simulink model "Partage_Simulink_2013"  (Simulink 8.2)
settings: Solver=ode5  SolverMode=SingleTasking  StartTime=0.0  StopTime=Smax/v-1  FixedStep=0.02  RelTol=1e-3
values from neighbouring files (symbols this model uses):
  A = eye(3) + A*Ts    [funcDriverModelAblamvi.m]    (also in funcDriverModelLoauy.m; funcNeuromuscularModel.m; funcTwoPointsVisualModel.m)
  alpha = 0.6    [Tref_combined.m]
  Aw = [-1/tau   1/tau ... (first row only)    [Tref_combined.m]
  Bs = 5.7    [Tref_combined.m]
  C = [       0       0       1       ]    [funcDriverModelAblamvi.m]    (also in funcDriverModelLoauy.m = zeros(2,3); funcNeuromuscularModel.m = zeros(1,1); funcTwoPointsVisualModel.m = zeros(1,2))
  Cw = [1  0]    [Tref_combined.m]
  EX0 = route.EX0    [Tref_combined.m]
  EY0 = route.EY0    [Tref_combined.m]
  F = A11d-L1*A21d    [Tref_combined.m]
  G = F*L1+A12d-L1*A22d    [Tref_combined.m]
  H = B1d-L1*B2d    [Tref_combined.m]
  Is = 0.05    [Tref_combined.m]
  Kplus_deltad = polyfit(alpha_vec,Kplus_vec(4,:),6)    [Tref_combined.m]
  Kplus_psiL = polyfit(alpha_vec,Kplus_vec(2,:),6)    [Tref_combined.m]
  Kplus_r = polyfit(alpha_vec,Kplus_vec(1,:),6)    [Tref_combined.m]
  Kplus_yL = polyfit(alpha_vec,Kplus_vec(3,:),7)    [Tref_combined.m]
  L1 = place(A11d',A21d',3*P0)'    [Tref_combined.m]
  Lo = acker(Aw',Cw',3*E)'    [Tref_combined.m]
  sw_DR = 1    [Tref_combined.m]
  sw_LQ = 0    [Tref_combined.m]
  T_horizon = 2    [Tref_combined.m]
  v = 18    [DriverModelLouayEstimationByPEM.m]    (also in NeuromuscularModelEstimationByPEM.m = 17; ParameterEstimationByPEM.m; Tref_combined.m; TwoPointsVisualModelEstimationByPEM.m = 17)
undefined symbols (not defined in the file or in its folder): Abic, Ad, At, Avr, B1, B1t, B2, B2t, Bbic, Bd, Bvr, Cbic, Cvr, D2, Dbic, Dvr, EPHI0, F2_a, fai_0_a, fai_2T8_a, fai_3T8_a, fai_4T8_a, fai_5T8_a, fai_6T8_a, fai_7T8_a, fai_T8_a, fai_T_a, Kplus_a, Measure, Measure_combined
libraries: simulink x2
settings Model: Creator=user  LastModifiedBy=Yishen Zhao
settings OptimizationCC: InitFltsAndDblsToZero=on
settings DebuggingCC: SaveWithParameterizedLinksMsg=none  SignalResolutionControl=TryResolveAllWithWarning  SolverPrmCheckMsg=none  MultiTaskDSMMsg=warning  MultiTaskCondExecSysMsg=none  FcnCallInpInsideContextMsg=EnableAllAsWarning  FrameProcessingCompatibilityMsg=error
settings GRTTargetCC: TargetFcnLib=ansi_tfl_tmw.mat  CodeReplacementLibrary=C89/C90 (ANSI)

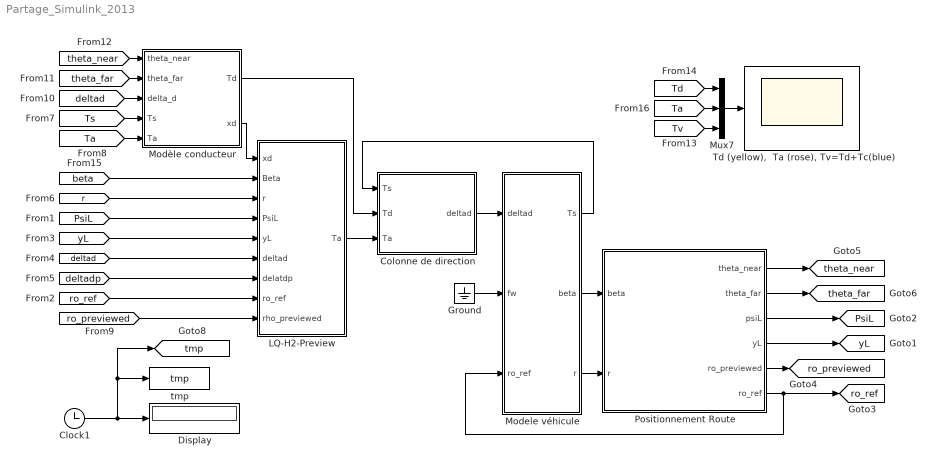
== system Partage_Simulink_2013 ==
  Clock1 : Clock
      settings: Decimation=60
  Colonne de direction : Subsystem
  Display : Display
  Ground : Ground
  LQ-H2-Preview : Subsystem
  Modele véhicule : Subsystem
  Modèle conducteur : Subsystem
  Mux7 : Mux  Inputs=3
  Positionnement Route : Subsystem  mask(Calcul des coordonnées x et y){}
      mask Display: disp('Calcul des coordonnées')
  "Td (yellow),  Ta (rose), Tv=Td+Tc(blue)" : Scope
      settings: TimeRange=auto  MaxDataPoints=5000  SaveName=TdTcTv  YMin=-20  YMax=15  SampleTime=-1
  tmp : ToWorkspace  VariableName=tmp  SampleTime=-1
  tag scope: PsiL=global, ro_previewed=global, ro_ref=global, theta_far=global, theta_near=global, tmp=global, yL=global
  wires:
  Clock1/1 -> Display/1, tmp/1, [tmp]
  Modele véhicule/3(r) -> Positionnement Route/2(r)
  Colonne de direction/1(deltad) -> Modele véhicule/1(deltad)
  Positionnement Route/6(ro_ref) -> [ro_ref], Modele véhicule/3(ro_ref)
  [r] -> LQ-H2-Preview/3(r)
  [PsiL] -> LQ-H2-Preview/4(PsiL)
  [yL] -> LQ-H2-Preview/5(yL)
  [deltad] -> LQ-H2-Preview/6(deltad)
  [deltadp] -> LQ-H2-Preview/7(delatdp)
  [ro_ref] -> LQ-H2-Preview/8(ro_ref)
  Positionnement Route/5(ro_previewed) -> [ro_previewed]
  Positionnement Route/1(theta_near) -> [theta_near]
  Positionnement Route/2(theta_far) -> [theta_far]
  [deltad] -> Modèle conducteur/3(delta_d)
  Positionnement Route/4(yL) -> [yL]
  Positionnement Route/3(psiL) -> [PsiL]
  Modele véhicule/2(beta) -> Positionnement Route/1(beta)
  Modele véhicule/1(Ts) -> Colonne de direction/1(Ts)
  [beta] -> LQ-H2-Preview/2(Beta)
  Modèle conducteur/2(xd) -> LQ-H2-Preview/1(xd)
  Mux7/1 -> "Td (yellow),  Ta (rose), Tv=Td+Tc(blue)"/1
  [theta_near] -> Modèle conducteur/1(theta_near)
  [Ts] -> Modèle conducteur/4(Ts)
  [Ta] -> Modèle conducteur/5(Ta)
  [theta_far] -> Modèle conducteur/2(theta_far)
  Ground/1 -> Modele véhicule/2(fw)
  [Td] -> Mux7/1
  [Ta] -> Mux7/2
  [Tv] -> Mux7/3
  Modèle conducteur/1(Td) -> Colonne de direction/2(Td)
  LQ-H2-Preview/1(Ta) -> Colonne de direction/3(Ta)
  [ro_previewed] -> LQ-H2-Preview/9(rho_previewed)

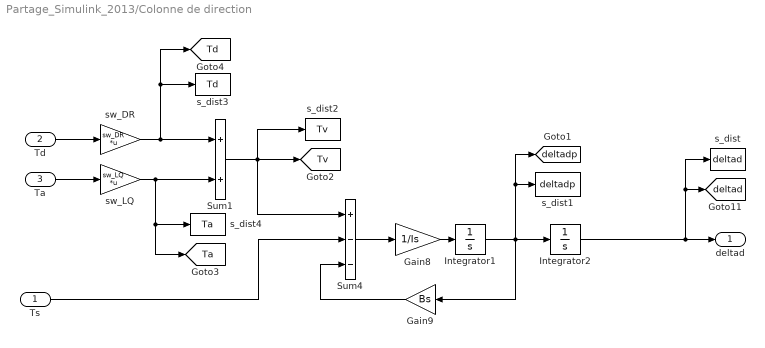
== system Partage_Simulink_2013/Colonne de direction ==
  Ts : Inport
  Td : Inport  Port=2
  Ta : Inport  Port=3
  Gain8 : Gain  Gain=1/Is  SaturateOnIntegerOverflow=on  OutDataTypeStr=Inherit: Same as input  ParamDataTypeStr=Inherit: Same as input
  Gain9 : Gain  Gain=Bs  SaturateOnIntegerOverflow=on  OutDataTypeStr=Inherit: Same as input  ParamDataTypeStr=Inherit: Same as input
  Integrator1 : Integrator
  Integrator2 : Integrator
  Sum1 : Sum  SaturateOnIntegerOverflow=on  InputSameDT=on  OutDataTypeStr=Inherit: Same as first input
  Sum4 : Sum  Inputs=+--  SaturateOnIntegerOverflow=on  InputSameDT=on  OutDataTypeStr=Inherit: Same as first input
  s_dist : ToWorkspace  VariableName=deltad  SampleTime=-1
  s_dist1 : ToWorkspace  VariableName=deltadp  SampleTime=-1
  s_dist2 : ToWorkspace  VariableName=Tv  SampleTime=-1
  s_dist3 : ToWorkspace  VariableName=Td  SampleTime=-1
  s_dist4 : ToWorkspace  VariableName=Ta  SampleTime=-1
  sw_DR : Gain  Gain=sw_DR  Multiplication=Matrix(K*u)  SaturateOnIntegerOverflow=on  OutDataTypeStr=Inherit: Same as input  ParamDataTypeStr=Inherit: Same as input
  sw_LQ : Gain  Gain=sw_LQ  Multiplication=Matrix(K*u)  SaturateOnIntegerOverflow=on  OutDataTypeStr=Inherit: Same as input  ParamDataTypeStr=Inherit: Same as input
  deltad : Outport
  tag scope: Ta=global, Td=global, Tv=global, deltad=global, deltadp=global
  wires:
  Gain8/1 -> Integrator1/1
  Sum4/1 -> Gain8/1
  Integrator1/1 -> Integrator2/1, s_dist1/1, [deltadp], Gain9/1
  Integrator2/1 -> deltad/1, [deltad], s_dist/1
  Ta/1 -> sw_LQ/1
  Gain9/1 -> Sum4/3
  Td/1 -> sw_DR/1
  sw_DR/1 -> Sum1/1, s_dist3/1, [Td]
  Ts/1 -> Sum4/2
  Sum1/1 -> Sum4/1, [Tv], s_dist2/1
  sw_LQ/1 -> s_dist4/1, [Ta], Sum1/2

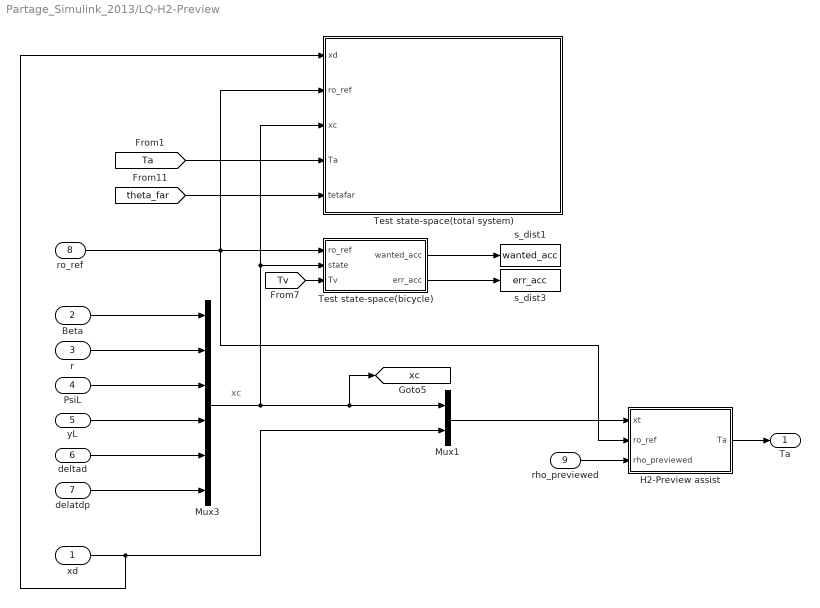
== system Partage_Simulink_2013/LQ-H2-Preview ==
  note: xc
  xd : Inport
  Beta : Inport  Port=2
  r : Inport  Port=3
  PsiL : Inport  Port=4
  yL : Inport  Port=5
  deltad : Inport  Port=6
  delatdp : Inport  Port=7
  ro_ref : Inport  Port=8
  rho_previewed : Inport  Port=9
  H2-Preview assist : Subsystem
  Mux1 : Mux  Inputs=2
  Mux3 : Mux  Inputs=6
  "Test state-space(bicycle) " : Subsystem
  Test state-space(total system) : Subsystem
  s_dist1 : ToWorkspace  VariableName=wanted_acc  SampleTime=-1
  s_dist3 : ToWorkspace  VariableName=err_acc  SampleTime=-1
  Ta : Outport
  tag scope: xc=global
  wires:
  Mux3/1 -> Test state-space(total system)/3(xc), "Test state-space(bicycle) "/2(state), [xc], Mux1/1
  Beta/1 -> Mux3/1
  r/1 -> Mux3/2
  PsiL/1 -> Mux3/3
  yL/1 -> Mux3/4
  deltad/1 -> Mux3/5
  delatdp/1 -> Mux3/6
  "Test state-space(bicycle) "/1(wanted_acc) -> s_dist1/1
  "Test state-space(bicycle) "/2(err_acc) -> s_dist3/1
  [Tv] -> "Test state-space(bicycle) "/3(Tv)
  [theta_far] -> Test state-space(total system)/5(tetafar)
  xd/1 -> Test state-space(total system)/1(xd), Mux1/2
  ro_ref/1 -> H2-Preview assist/2("ro_ref "), "Test state-space(bicycle) "/1(ro_ref), Test state-space(total system)/2(ro_ref)
  Mux1/1 -> H2-Preview assist/1(xt)
  [Ta] -> Test state-space(total system)/4(Ta)
  H2-Preview assist/1(Ta) -> Ta/1
  rho_previewed/1 -> H2-Preview assist/3(rho_previewed)

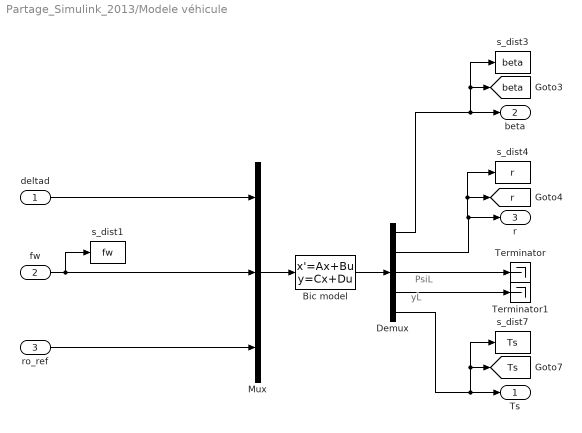
== system Partage_Simulink_2013/Modele véhicule ==
  note: PsiL
  note: yL
  deltad : Inport
  fw : Inport  Port=2
  ro_ref : Inport  Port=3
  Bic model : StateSpace  A=Abic  B=Bbic  C=Cbic  D=Dbic  X0=[0;0;0;0]
  Demux : Demux  Outputs=5
  Mux : Mux  Inputs=3
  Terminator : Terminator
  Terminator1 : Terminator
  s_dist1 : ToWorkspace  VariableName=fw  SampleTime=-1
  s_dist3 : ToWorkspace  VariableName=beta  SampleTime=-1
  s_dist4 : ToWorkspace  VariableName=r  SampleTime=-1
  s_dist7 : ToWorkspace  VariableName=Ts  SampleTime=-1
  Ts : Outport
  beta : Outport  Port=2
  r : Outport  Port=3
  tag scope: Ts=global, beta=global, r=global
  wires:
  fw/1 -> Mux/2, s_dist1/1
  ro_ref/1 -> Mux/3
  Mux/1 -> Bic model/1
  Bic model/1 -> Demux/1
  deltad/1 -> Mux/1
  Demux/1 -> beta/1, [beta], s_dist3/1
  Demux/2 -> s_dist4/1, [r], r/1
  Demux/5 -> Ts/1, [Ts], s_dist7/1
  Demux/3 -> Terminator/1
  Demux/4 -> Terminator1/1

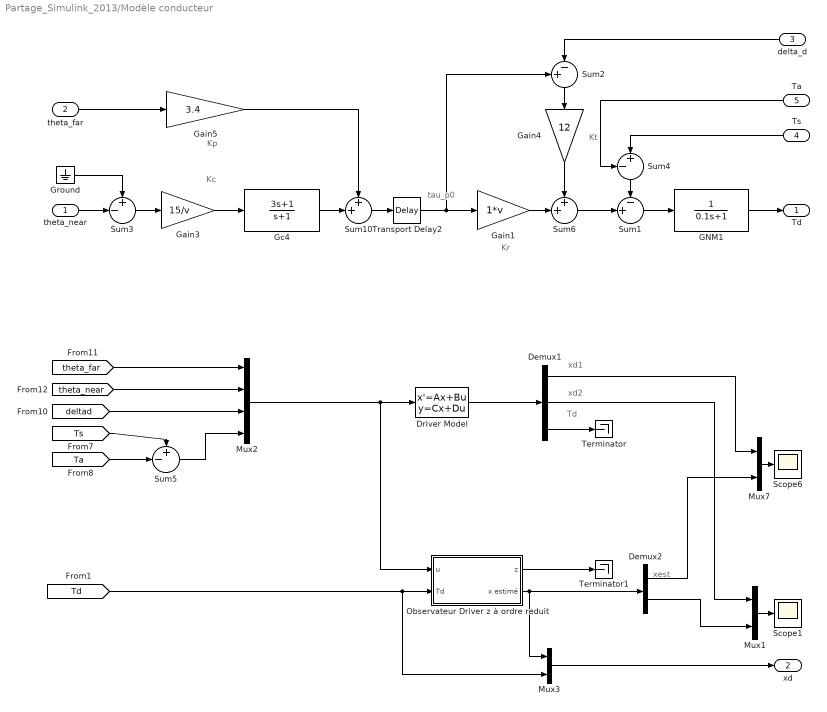
== system Partage_Simulink_2013/Modèle conducteur ==
  note: Kc
  note: tau_p0
  note: Kr
  note: Kp
  note: Kt
  note: xd1
  note: xd2
  note: Td
  note: xest
  theta_near : Inport
  theta_far : Inport  Port=2
  delta_d : Inport  Port=3
  Ts : Inport  Port=4
  Ta : Inport  Port=5
  Demux1 : Demux  Outputs=3
  Demux2 : Demux  Outputs=2
  Driver Model : StateSpace  A=Ad  B=Bd  C=[1 0 0;0 1 0;0 0 1]  D=[0 0 0 0;0 0 0 0;0 0 0 0]  X0=[0;0;0]
  GNM1 : TransferFcn  Numerator=1  Denominator=[0.1 1]
  Gain1 : Gain  Gain=1*v  SaturateOnIntegerOverflow=on  OutDataTypeStr=Inherit: Same as input  ParamDataTypeStr=Inherit: Same as input
  Gain3 : Gain  Gain=15/v  SaturateOnIntegerOverflow=on  OutDataTypeStr=Inherit: Same as input  ParamDataTypeStr=Inherit: Same as input
  Gain4 : Gain  Gain=12  SaturateOnIntegerOverflow=on  OutDataTypeStr=Inherit: Same as input  ParamDataTypeStr=Inherit: Same as input
  Gain5 : Gain  Gain=3.4  SaturateOnIntegerOverflow=on  OutDataTypeStr=Inherit: Same as input  ParamDataTypeStr=Inherit: Same as input
  Gc4 : TransferFcn  Numerator=[3 1]  Denominator=[1 1]
  Ground : Ground
  Mux1 : Mux  Inputs=2
  Mux2 : Mux
  Mux3 : Mux  Inputs=2
  Mux7 : Mux  Inputs=2
  Observateur Driver z à ordre reduit : Subsystem
  Scope1 : Scope
      settings: TimeRange=auto  LimitDataPoints=on  MaxDataPoints=5000  SaveToWorkspace=off  SaveName=ScopeData9  YMin=-8  YMax=7  SampleTime=-1
  Scope6 : Scope
      settings: TimeRange=auto  LimitDataPoints=on  MaxDataPoints=5000  SaveToWorkspace=off  SaveName=ScopeData8  YMin=-0.15  YMax=0.2  SampleTime=-1
  Sum1 : Sum  Inputs=-+|  SaturateOnIntegerOverflow=on  InputSameDT=on  OutDataTypeStr=Inherit: Same as first input
  Sum10 : Sum  Inputs=++|  SaturateOnIntegerOverflow=on  InputSameDT=on  OutDataTypeStr=Inherit: Same as first input
  Sum2 : Sum  Inputs=+-|  SaturateOnIntegerOverflow=on  InputSameDT=on  OutDataTypeStr=Inherit: Same as first input
  Sum3 : Sum  Inputs=+-|  SaturateOnIntegerOverflow=on  InputSameDT=on  OutDataTypeStr=Inherit: Same as first input
  Sum4 : Sum  Inputs=-+|  SaturateOnIntegerOverflow=on  InputSameDT=on  OutDataTypeStr=Inherit: Same as first input
  Sum5 : Sum  Inputs=+-|  SaturateOnIntegerOverflow=on  InputSameDT=on  OutDataTypeStr=Inherit: Same as first input
  Sum6 : Sum  Inputs=++|  SaturateOnIntegerOverflow=on  InputSameDT=on  OutDataTypeStr=Inherit: Same as first input
  Terminator : Terminator
  Terminator1 : Terminator
  Transport Delay2 : TransportDelay  DelayTime=0.04
  Td : Outport
  xd : Outport  Port=2
  wires:
  theta_far/1 -> Gain5/1
  theta_near/1 -> Sum3/2
  Ground/1 -> Sum3/1
  Gain5/1 -> Sum10/1
  Sum3/1 -> Gain3/1
  Sum1/1 -> GNM1/1
  Gain3/1 -> Gc4/1
  Gc4/1 -> Sum10/2
  Sum10/1 -> Transport Delay2/1
  Transport Delay2/1 -> Sum2/1, Gain1/1
  Gain1/1 -> Sum6/2
  delta_d/1 -> Sum2/2
  Sum2/1 -> Gain4/1
  Gain4/1 -> Sum6/1
  Driver Model/1 -> Demux1/1
  [theta_near] -> Mux2/2
  [deltad] -> Mux2/3
  GNM1/1 -> Td/1
  Sum6/1 -> Sum1/2
  Sum5/1 -> Mux2/4
  [Ta] -> Sum5/2
  [Ts] -> Sum5/1
  Sum4/1 -> Sum1/1
  Ts/1 -> Sum4/2
  Ta/1 -> Sum4/1
  [theta_far] -> Mux2/1
  Observateur Driver z à ordre reduit/2(x estimé) -> Demux2/1, Mux3/1
  Mux7/1 -> Scope6/1
  Demux1/1 -> Mux7/1
  Demux2/1 -> Mux7/2
  Mux1/1 -> Scope1/1
  Demux1/2 -> Mux1/1
  Demux2/2 -> Mux1/2
  [Td] -> Observateur Driver z à ordre reduit/2(Td), Mux3/2
  Mux2/1 -> Driver Model/1, Observateur Driver z à ordre reduit/1(u)
  Mux3/1 -> xd/1
  Demux1/3 -> Terminator/1
  Observateur Driver z à ordre reduit/1(z) -> Terminator1/1

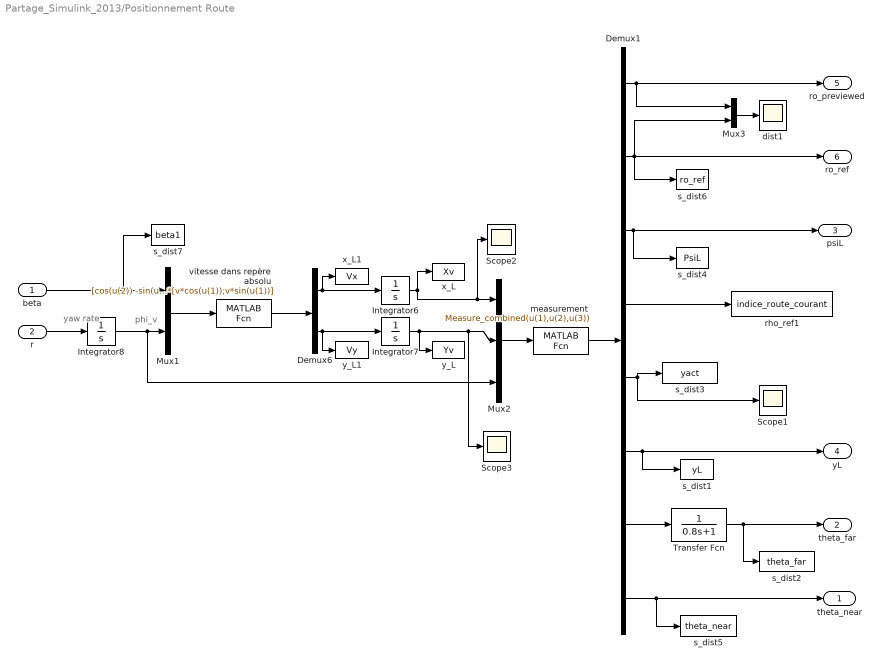
== system Partage_Simulink_2013/Positionnement Route ==
  note: phi_v
  note: yaw rate
  beta : Inport
  r : Inport  Port=2
  Demux1 : Demux  Outputs=8
  Demux6 : Demux  Outputs=2
  Integrator6 : Integrator  InitialCondition=EX0
  Integrator7 : Integrator  InitialCondition=EY0
  Integrator8 : Integrator  InitialCondition=EPHI0
  Mux1 : Mux  Inputs=2
  Mux2 : Mux  Inputs=3
  Mux3 : Mux  Inputs=2
  Scope1 : Scope
      settings: TimeRange=auto  LimitDataPoints=on  MaxDataPoints=5000  SaveToWorkspace=off  SaveName=ScopeData7  YMin=-4.92978  YMax=4.87495  SampleTime=-1
  Scope2 : Scope
      settings: TimeRange=auto  LimitDataPoints=on  MaxDataPoints=5000  SaveToWorkspace=off  SaveName=ScopeData18  YMin=-967.24148  YMax=375.02741  SampleTime=-1
  Scope3 : Scope
      settings: TimeRange=auto  LimitDataPoints=on  MaxDataPoints=5000  SaveToWorkspace=off  SaveName=ScopeData19  YMin=-10  YMax=10  SampleTime=-1
  Transfer Fcn : TransferFcn  Denominator=[0.8 1]
  dist1 : Scope
      settings: TimeRange=auto  MaxDataPoints=5000  SaveToWorkspace=off  SaveName=ScopeData10  YMin=-0.03  YMax=0.04  SampleTime=-1
  measurement : MATLABFcn  MATLABFcn=Measure_combined(u(1),u(2),u(3))  OutputDimensions=8
  rho_ref1 : ToWorkspace  VariableName=indice_route_courant  SampleTime=-1
  s_dist1 : ToWorkspace  VariableName=yL  SampleTime=-1
  s_dist2 : ToWorkspace  VariableName=theta_far  SampleTime=-1
  s_dist3 : ToWorkspace  VariableName=yact  SampleTime=-1
  s_dist4 : ToWorkspace  VariableName=PsiL  SampleTime=-1
  s_dist5 : ToWorkspace  VariableName=theta_near  SampleTime=-1
  s_dist6 : ToWorkspace  VariableName=ro_ref  SampleTime=-1
  s_dist7 : ToWorkspace  VariableName=beta1  SampleTime=-1
  vitesse dans repère absolu : MATLABFcn  MATLABFcn=[cos(u(2)) -sin(u(2));sin(u(2)) cos(u(2)) ]*[v*cos(u(1));v*sin(u(1))]  OutputDimensions=2
  x_L : ToWorkspace  VariableName=Xv  SampleTime=-1
  x_L1 : ToWorkspace  VariableName=Vx  SampleTime=-1
  y_L : ToWorkspace  VariableName=Yv  SampleTime=-1
  y_L1 : ToWorkspace  VariableName=Vy  SampleTime=-1
  theta_near : Outport
  theta_far : Outport  Port=2
  psiL : Outport  Port=3
  yL : Outport  Port=4
  ro_previewed : Outport  Port=5
  ro_ref : Outport  Port=6
  wires:
  vitesse dans repère absolu/1 -> Demux6/1
  Integrator8/1 -> Mux1/2, Mux2/3
  Mux1/1 -> vitesse dans repère absolu/1
  Demux6/1 -> Integrator6/1, x_L1/1
  Demux6/2 -> y_L1/1, Integrator7/1
  Integrator6/1 -> Scope2/1, Mux2/1, x_L/1
  Integrator7/1 -> Scope3/1, Mux2/2, y_L/1
  Mux2/1 -> measurement/1
  r/1 -> Integrator8/1
  Demux1/1 -> ro_previewed/1, Mux3/1
  Demux1/2 -> ro_ref/1, s_dist6/1, Mux3/2
  measurement/1 -> Demux1/1
  Demux1/4 -> rho_ref1/1
  Demux1/5 -> s_dist3/1, Scope1/1
  Demux1/8 -> s_dist5/1, theta_near/1
  Demux1/7 -> Transfer Fcn/1
  Demux1/3 -> s_dist4/1, psiL/1
  Demux1/6 -> s_dist1/1, yL/1
  Transfer Fcn/1 -> s_dist2/1, theta_far/1
  Mux3/1 -> dist1/1
  beta/1 -> s_dist7/1, Mux1/1

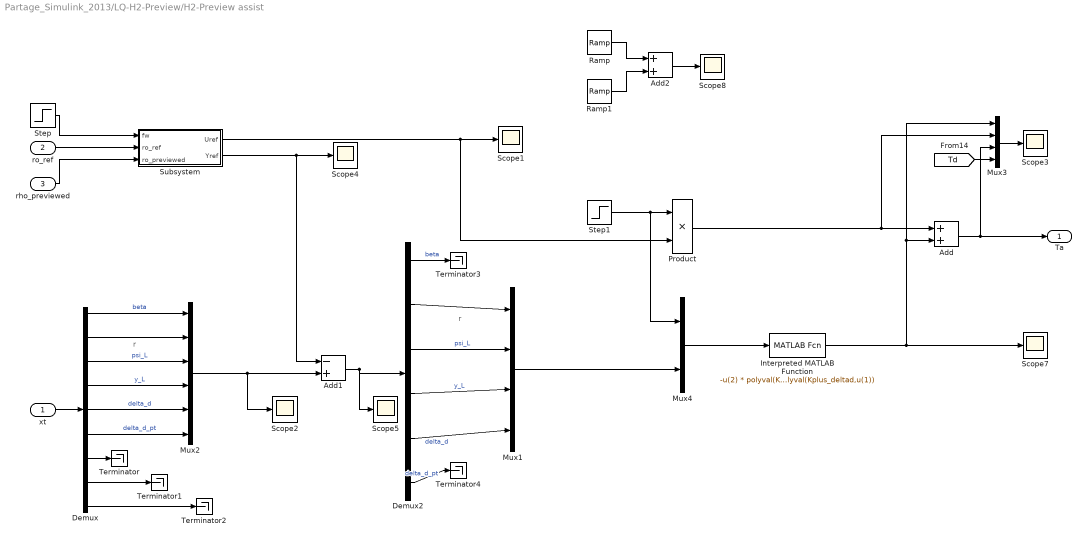
== system Partage_Simulink_2013/LQ-H2-Preview/H2-Preview assist ==
  note: r
  note: r
  xt : Inport
  "ro_ref " : Inport  Port=2
  rho_previewed : Inport  Port=3
  Add : Sum
  Add1 : Sum  Inputs=-+
  Add2 : Sum
  Demux : Demux  Outputs=9
  Demux2 : Demux  Outputs=6
  Interpreted MATLAB Function : MATLABFcn  MATLABFcn="-u(2) * polyval(Kplus_r,u(1))-  u(3) * polyval(Kplus_psiL,u(1)) -  u(4) * polyval(Kplus_yL,u(1))  - u(5) * polyval(Kplus_deltad,u(1))"  OutputDimensions=1
  Mux1 : Mux
  Mux2 : Mux  Inputs=6
  Mux3 : Mux
  Mux4 : Mux  Inputs=2
  Product : Product
  Ramp : simulink/Sources/Ramp  slope=-0.05  start=70  X0=0
  Ramp1 : simulink/Sources/Ramp  slope=0.05  start=50  X0=0
  Scope{1..5,7..8} (7 alike) : Scope
      Scope1 settings: TimeRange=auto  MaxDataPoints=5000  SaveToWorkspace=off  YMin=-13.36133  YMax=22.74481  SampleTime=-1
      Scope2 settings: TimeRange=auto  LimitDataPoints=on  MaxDataPoints=5000  SaveToWorkspace=off  SaveName=ScopeData16  YMin=-1.5452  YMax=1.78462  SampleTime=-1  DataFormat=Array
      Scope3 settings: TimeRange=auto  ShowLegends=on  MaxDataPoints=5000  SaveToWorkspace=off  SaveName=ScopeData17  YMin=-8.25778  YMax=15.55129  SampleTime=-1  DataFormat=Array
      Scope4 settings: TimeRange=auto  ShowLegends=on  MaxDataPoints=5000  SaveToWorkspace=off  SaveName=ScopeData2  YMin=-2.24568  YMax=2.40321  SampleTime=-1
      Scope5 settings: TimeRange=auto  ShowLegends=on  MaxDataPoints=5000  SaveToWorkspace=off  YMin=-1.38701  YMax=1.61243  SampleTime=-1  DataFormat=Array
      Scope7 settings: TimeRange=auto  MaxDataPoints=5000  SaveToWorkspace=off  SaveName=ScopeData4  YMin=-3.07143  YMax=4.24815  SampleTime=-1
      Scope8 settings: TimeRange=auto  MaxDataPoints=5000  SaveToWorkspace=off  YMin=-0.125  YMax=1.125  SampleTime=-1
  Step : Step  After=0  SampleTime=0
  Step1 : Step  Before=alpha  After=alpha  SampleTime=0
  Subsystem : Subsystem
  Terminator{,1..4} (5 alike) : Terminator
  Ta : Outport
  wires:
  xt/1 -> Demux/1
  Demux/1 -> Mux2/1  "beta"
  Demux/2 -> Mux2/2
  Demux/3 -> Mux2/3  "psi_L"
  Demux/4 -> Mux2/4  "y_L"
  Demux/5 -> Mux2/5  "delta_d"
  Demux/6 -> Mux2/6  "delta_d_pt"
  Mux2/1 -> Scope2/1, Add1/2
  Add/1 -> Mux3/3, Ta/1
  Interpreted MATLAB Function/1 -> Mux3/1, Add/2, Scope7/1
  Demux/7 -> Terminator/1
  Demux/8 -> Terminator1/1
  Demux/9 -> Terminator2/1
  Subsystem/2(Yref) -> Add1/1, Scope4/1
  Subsystem/1(Uref) -> Product/2, Scope1/1
  Step/1 -> Subsystem/1("fw ")
  rho_previewed/1 -> Subsystem/3(ro_previewed)
  "ro_ref "/1 -> Subsystem/2("ro_ref ")
  Product/1 -> Mux3/2, Add/1
  Add1/1 -> Scope5/1, Demux2/1
  Demux2/2 -> Mux1/1
  Demux2/3 -> Mux1/2  "psi_L"
  Demux2/4 -> Mux1/3  "y_L"
  Demux2/5 -> Mux1/4  "delta_d"
  Mux3/1 -> Scope3/1
  Demux2/1 -> Terminator3/1  "beta"
  Demux2/6 -> Terminator4/1  "delta_d_pt"
  Add2/1 -> Scope8/1
  Mux1/1 -> Mux4/2
  Mux4/1 -> Interpreted MATLAB Function/1
  Step1/1 -> Mux4/1, Product/1
  [Td] -> Mux3/4
  Ramp/1 -> Add2/1
  Ramp1/1 -> Add2/2

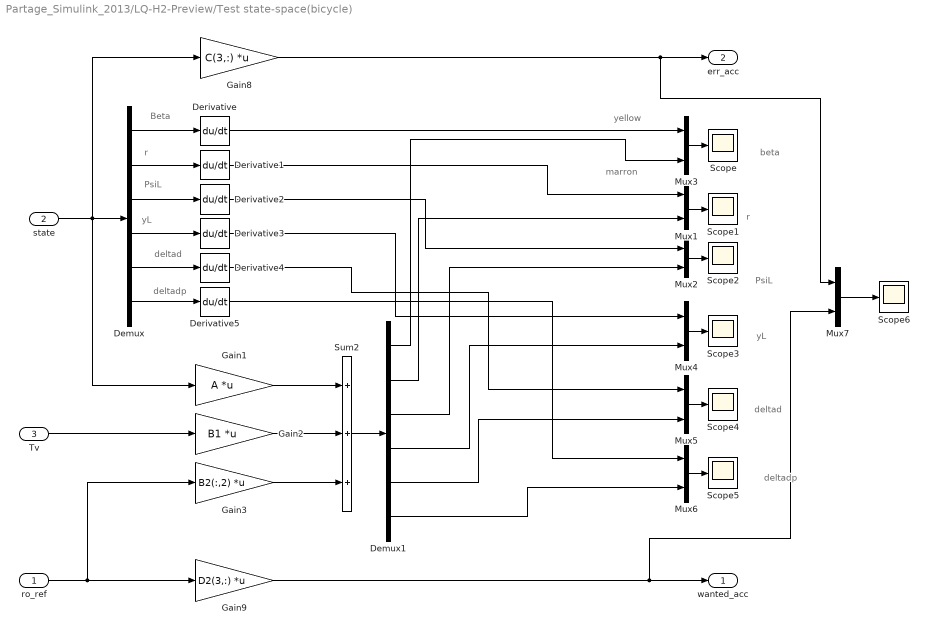
== system Partage_Simulink_2013/LQ-H2-Preview/Test state-space(bicycle)  ==
  note: Beta
  note: r
  note: PsiL
  note: yL
  note: deltad
  note: deltadp
  note: beta
  note: r
  note: PsiL
  note: yL
  note: deltad
  note: deltadp
  note: yellow
  note: marron
  ro_ref : Inport
  state : Inport  Port=2
  Tv : Inport  Port=3
  Demux : Demux  Outputs=6
  Demux1 : Demux  Outputs=6
  Derivative{,1..5} (6 alike) : Derivative
  Gain1 : Gain  Gain=A  Multiplication=Matrix(K*u)  SaturateOnIntegerOverflow=on  OutDataTypeStr=Inherit: Same as input  ParamDataTypeStr=Inherit: Same as input
  Gain2 : Gain  Gain=B1  Multiplication=Matrix(K*u)  SaturateOnIntegerOverflow=on  OutDataTypeStr=Inherit: Same as input  ParamDataTypeStr=Inherit: Same as input
  Gain3 : Gain  Gain=B2(:,2)  Multiplication=Matrix(K*u)  SaturateOnIntegerOverflow=on  OutDataTypeStr=Inherit: Same as input  ParamDataTypeStr=Inherit: Same as input
  Gain8 : Gain  Gain=C(3,:)  Multiplication=Matrix(K*u)  SaturateOnIntegerOverflow=on  OutDataTypeStr=Inherit: Same as input  ParamDataTypeStr=Inherit: Same as input
  Gain9 : Gain  Gain=D2(3,:)  Multiplication=Matrix(K*u)  SaturateOnIntegerOverflow=on  OutDataTypeStr=Inherit: Same as input  ParamDataTypeStr=Inherit: Same as input
  Mux{1..7} (7 alike) : Mux  Inputs=2
  Scope{,1..6} (7 alike) : Scope
      Scope settings: TimeRange=auto  LimitDataPoints=on  MaxDataPoints=5000  SaveToWorkspace=off  SaveName=ScopeData  YMin=-0.02686  YMax=0.02074  SampleTime=-1
      Scope1 settings: TimeRange=auto  LimitDataPoints=on  MaxDataPoints=5000  SaveToWorkspace=off  YMin=-0.44331  YMax=0.60512  SampleTime=-1
      Scope2 settings: TimeRange=auto  LimitDataPoints=on  MaxDataPoints=5000  SaveToWorkspace=off  SaveName=ScopeData2  YMin=-0.16868  YMax=0.17015  SampleTime=-1
      Scope3 settings: TimeRange=auto  LimitDataPoints=on  MaxDataPoints=5000  SaveToWorkspace=off  SaveName=ScopeData3  YMin=-1.19429  YMax=1.3221  SampleTime=-1
      Scope4 settings: TimeRange=auto  LimitDataPoints=on  MaxDataPoints=5000  SaveToWorkspace=off  SaveName=ScopeData4  YMin=-1.21005  YMax=1.63703  SampleTime=-1
      Scope5 settings: TimeRange=auto  LimitDataPoints=on  MaxDataPoints=5000  SaveToWorkspace=off  SaveName=ScopeData6  YMin=-77.88552  YMax=58.6837  SampleTime=-1
      Scope6 settings: TimeRange=auto  ShowLegends=on  LimitDataPoints=on  MaxDataPoints=5000  SaveToWorkspace=off  YMin=-9.19531  YMax=8.21466  SampleTime=-1
  Sum2 : Sum  Inputs=+++  SaturateOnIntegerOverflow=on  InputSameDT=on  OutDataTypeStr=Inherit: Same as first input
  wanted_acc : Outport
  err_acc : Outport  Port=2
  wires:
  state/1 -> Demux/1, Gain1/1, Gain8/1
  Gain9/1 -> Mux7/2, wanted_acc/1
  ro_ref/1 -> Gain9/1, Gain3/1
  Gain8/1 -> Mux7/1, err_acc/1
  Demux/1 -> Derivative/1
  Gain1/1 -> Sum2/1
  Gain2/1 -> Sum2/2
  Gain3/1 -> Sum2/3
  Sum2/1 -> Demux1/1
  Mux3/1 -> Scope/1
  Demux1/1 -> Mux3/2
  Demux/2 -> Derivative1/1
  Demux/3 -> Derivative2/1
  Demux/4 -> Derivative3/1
  Demux/5 -> Derivative4/1
  Demux/6 -> Derivative5/1
  Mux1/1 -> Scope1/1
  Mux2/1 -> Scope2/1
  Mux4/1 -> Scope3/1
  Derivative1/1 -> Mux1/1
  Demux1/2 -> Mux1/2
  Derivative3/1 -> Mux4/1
  Demux1/4 -> Mux4/2
  Mux5/1 -> Scope4/1
  Derivative4/1 -> Mux5/1
  Demux1/5 -> Mux5/2
  Mux6/1 -> Scope5/1
  Derivative5/1 -> Mux6/1
  Demux1/6 -> Mux6/2
  Derivative/1 -> Mux3/1
  Derivative2/1 -> Mux2/1
  Demux1/3 -> Mux2/2
  Tv/1 -> Gain2/1
  Mux7/1 -> Scope6/1

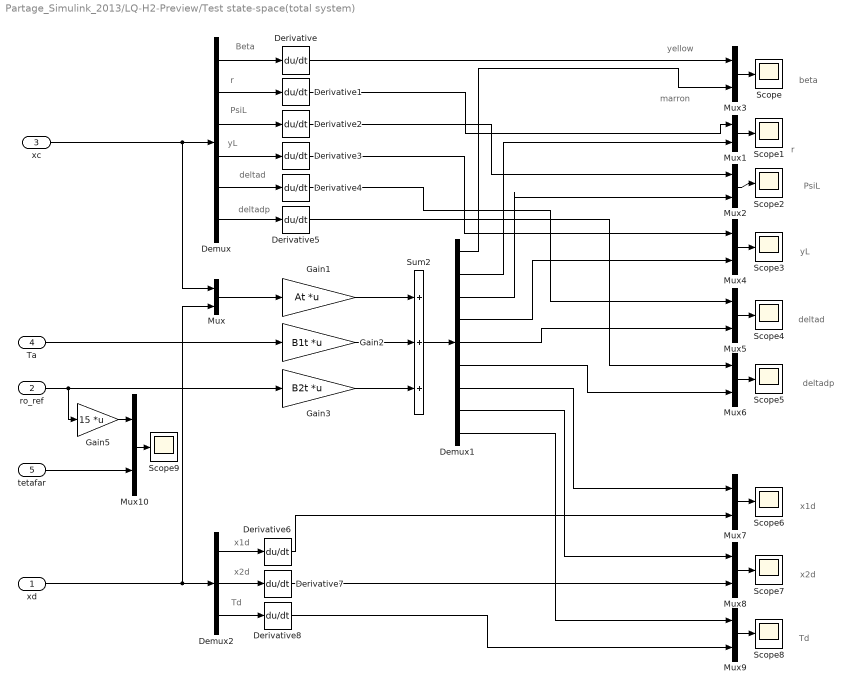
== system Partage_Simulink_2013/LQ-H2-Preview/Test state-space(total system) ==
  note: Beta
  note: r
  note: PsiL
  note: yL
  note: deltad
  note: deltadp
  note: beta
  note: r
  note: PsiL
  note: yL
  note: deltad
  note: deltadp
  note: yellow
  note: marron
  note: Td
  note: x1d
  note: x2d
  note: x1d
  note: x2d
  note: Td
  xd : Inport
  ro_ref : Inport  Port=2
  xc : Inport  Port=3  PortDimensions=6
  Ta : Inport  Port=4
  tetafar : Inport  Port=5
  Demux : Demux  Outputs=6
  Demux1 : Demux  Outputs=9
  Demux2 : Demux  Outputs=3
  Derivative{,1..8} (9 alike) : Derivative
  Gain1 : Gain  Gain=At  Multiplication=Matrix(K*u)  SaturateOnIntegerOverflow=on  OutDataTypeStr=Inherit: Same as input  ParamDataTypeStr=Inherit: Same as input
  Gain2 : Gain  Gain=B1t  Multiplication=Matrix(K*u)  SaturateOnIntegerOverflow=on  OutDataTypeStr=Inherit: Same as input  ParamDataTypeStr=Inherit: Same as input
  Gain3 : Gain  Gain=B2t  Multiplication=Matrix(K*u)  SaturateOnIntegerOverflow=on  OutDataTypeStr=Inherit: Same as input  ParamDataTypeStr=Inherit: Same as input
  Gain5 : Gain  Gain=15  Multiplication=Matrix(K*u)  SaturateOnIntegerOverflow=on  OutDataTypeStr=Inherit: Same as input  ParamDataTypeStr=Inherit: Same as input
  Mux{,1..10} (11 alike) : Mux  Inputs=2
  Scope{,1..9} (10 alike) : Scope
      Scope settings: TimeRange=auto  LimitDataPoints=on  MaxDataPoints=5000  SaveToWorkspace=off  SaveName=ScopeData  YMin=-10  YMax=10  SampleTime=-1
      Scope1 settings: TimeRange=auto  LimitDataPoints=on  MaxDataPoints=5000  SaveToWorkspace=off  YMin=-10  YMax=10  SampleTime=-1
      Scope2 settings: TimeRange=auto  LimitDataPoints=on  MaxDataPoints=5000  SaveToWorkspace=off  SaveName=ScopeData2  YMin=-10  YMax=10  SampleTime=-1
      Scope3 settings: TimeRange=auto  LimitDataPoints=on  MaxDataPoints=5000  SaveToWorkspace=off  SaveName=ScopeData3  YMin=-10  YMax=10  SampleTime=-1
      Scope4 settings: TimeRange=auto  LimitDataPoints=on  MaxDataPoints=5000  SaveToWorkspace=off  SaveName=ScopeData4  YMin=-10  YMax=10  SampleTime=-1
      Scope5 settings: TimeRange=auto  LimitDataPoints=on  MaxDataPoints=5000  SaveToWorkspace=off  SaveName=ScopeData6  YMin=-10  YMax=10  SampleTime=-1
      Scope6 settings: TimeRange=auto  LimitDataPoints=on  MaxDataPoints=5000  SaveToWorkspace=off  SaveName=ScopeData11  YMin=-10  YMax=10  SampleTime=-1
      Scope7 settings: TimeRange=auto  LimitDataPoints=on  MaxDataPoints=5000  SaveToWorkspace=off  SaveName=ScopeData12  YMin=-10  YMax=10  SampleTime=-1
      Scope8 settings: TimeRange=auto  LimitDataPoints=on  MaxDataPoints=5000  SaveToWorkspace=off  SaveName=ScopeData13  YMin=-10  YMax=10  SampleTime=-1
      Scope9 settings: TimeRange=auto  LimitDataPoints=on  MaxDataPoints=5000  SaveToWorkspace=off  SaveName=ScopeData14  YMin=-10  YMax=10  SampleTime=-1
  Sum2 : Sum  Inputs=+++  SaturateOnIntegerOverflow=on  InputSameDT=on  OutDataTypeStr=Inherit: Same as first input
  wires:
  xc/1 -> Demux/1, Mux/1
  ro_ref/1 -> Gain5/1, Gain3/1
  Demux/1 -> Derivative/1
  Gain1/1 -> Sum2/1
  Gain2/1 -> Sum2/2
  Gain3/1 -> Sum2/3
  Sum2/1 -> Demux1/1
  Mux3/1 -> Scope/1
  Demux1/1 -> Mux3/2
  Demux/2 -> Derivative1/1
  Demux/3 -> Derivative2/1
  Demux/4 -> Derivative3/1
  Demux/5 -> Derivative4/1
  Demux/6 -> Derivative5/1
  Mux1/1 -> Scope1/1
  Mux2/1 -> Scope2/1
  Mux4/1 -> Scope3/1
  Derivative1/1 -> Mux1/1
  Demux1/2 -> Mux1/2
  Derivative3/1 -> Mux4/1
  Demux1/4 -> Mux4/2
  Mux5/1 -> Scope4/1
  Derivative4/1 -> Mux5/1
  Demux1/5 -> Mux5/2
  Mux6/1 -> Scope5/1
  Derivative5/1 -> Mux6/1
  Demux1/6 -> Mux6/2
  Derivative/1 -> Mux3/1
  Derivative2/1 -> Mux2/1
  Demux1/3 -> Mux2/2
  Ta/1 -> Gain2/1
  xd/1 -> Demux2/1, Mux/2
  Demux2/1 -> Derivative6/1
  Demux2/2 -> Derivative7/1
  Demux2/3 -> Derivative8/1
  Mux/1 -> Gain1/1
  Mux7/1 -> Scope6/1
  Mux8/1 -> Scope7/1
  Mux9/1 -> Scope8/1
  Demux1/7 -> Mux7/1
  Demux1/8 -> Mux8/1
  Demux1/9 -> Mux9/1
  Derivative6/1 -> Mux7/2
  Derivative7/1 -> Mux8/2
  Derivative8/1 -> Mux9/2
  Gain5/1 -> Mux10/1
  Mux10/1 -> Scope9/1
  tetafar/1 -> Mux10/2

== system Partage_Simulink_2013/Modèle conducteur/Observateur Driver z à ordre reduit ==
  note: z
  u : Inport
  Td : Inport  Port=2
  F : Gain  Gain=F  Multiplication=Matrix(K*u)  SaturateOnIntegerOverflow=on  OutDataTypeStr=Inherit: Same as input  ParamDataTypeStr=Inherit: Same as input
  G : Gain  Gain=G  Multiplication=Matrix(K*u)  SaturateOnIntegerOverflow=on  OutDataTypeStr=Inherit: Same as input  ParamDataTypeStr=Inherit: Same as input
  H : Gain  Gain=H  Multiplication=Matrix(K*u)  SaturateOnIntegerOverflow=on  OutDataTypeStr=Inherit: Same as input  ParamDataTypeStr=Inherit: Same as input
  Integrator1 : Integrator
  Ld : Gain  Gain=L1  Multiplication=Matrix(K*u)  SaturateOnIntegerOverflow=on  OutDataTypeStr=Inherit: Same as input  ParamDataTypeStr=Inherit: Same as input
  Sum7 : Sum  Inputs=+++  SaturateOnIntegerOverflow=on  InputSameDT=on  OutDataTypeStr=Inherit: Same as first input
  Sum8 : Sum  SaturateOnIntegerOverflow=on  InputSameDT=on  OutDataTypeStr=Inherit: Same as first input
  z : Outport
  x estimé : Outport  Port=2
  wires:
  u/1 -> H/1
  Integrator1/1 -> F/1, Sum8/1, z/1
  Sum7/1 -> Integrator1/1
  F/1 -> Sum7/3
  H/1 -> Sum7/1
  G/1 -> Sum7/2
  Td/1 -> Ld/1, G/1
  Ld/1 -> Sum8/2
  Sum8/1 -> x estimé/1

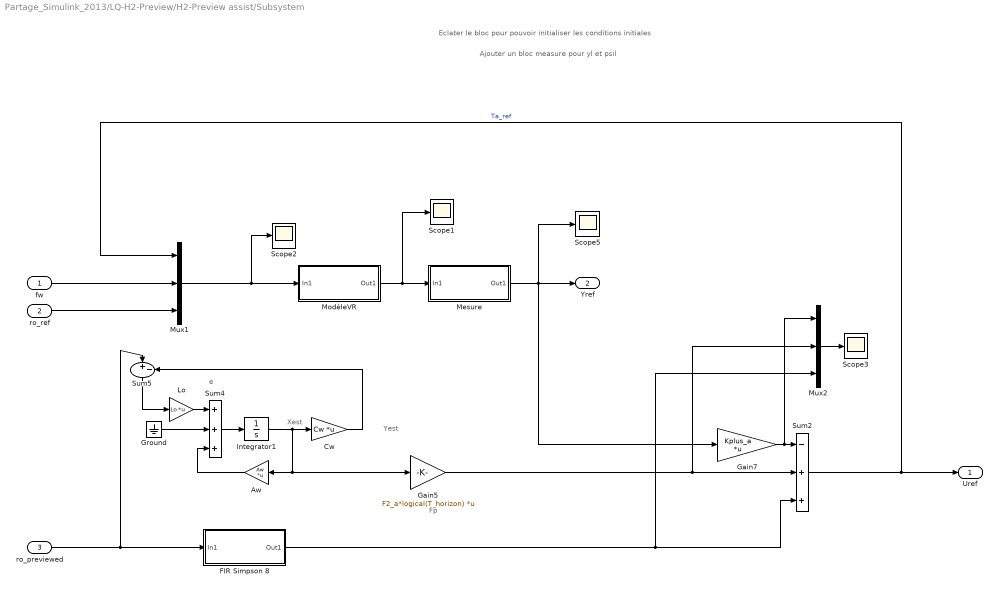
== system Partage_Simulink_2013/LQ-H2-Preview/H2-Preview assist/Subsystem ==
  note: Eclater le bloc pour pouvoir initialiser les conditions initiales
  note: Ajouter un bloc measure pour yl et psil
  note: Yest
  note: e
  note: Xest
  note: Fp
  "fw " : Inport
  "ro_ref " : Inport  Port=2
  ro_previewed : Inport  Port=3
  Aw : Gain  Gain=Aw  Multiplication=Matrix(K*u)  SaturateOnIntegerOverflow=on  OutDataTypeStr=Inherit: Same as input  ParamDataTypeStr=Inherit: Same as input
  Cw : Gain  Gain=Cw  Multiplication=Matrix(K*u)  SaturateOnIntegerOverflow=on  OutDataTypeStr=Inherit: Same as input  ParamDataTypeStr=Inherit: Same as input
  FIR Simpson 8 : Subsystem
  Gain5 : Gain  Gain=F2_a*logical(T_horizon)  Multiplication=Matrix(K*u)  SaturateOnIntegerOverflow=on  OutDataTypeStr=Inherit: Same as input  ParamDataTypeStr=Inherit: Same as input
  Gain7 : Gain  Gain=Kplus_a  Multiplication=Matrix(K*u)  SaturateOnIntegerOverflow=on  OutDataTypeStr=Inherit: Same as input  ParamDataTypeStr=Inherit: Same as input
  Ground : Ground
  Integrator1 : Integrator
  Lo : Gain  Gain=Lo  Multiplication=Matrix(K*u)  SaturateOnIntegerOverflow=on  OutDataTypeStr=Inherit: Same as input  ParamDataTypeStr=Inherit: Same as input
  Mesure : Subsystem
  ModèleVR : Subsystem
  Mux1 : Mux  Inputs=3
  Mux2 : Mux  Inputs=3
  Scope{1..3,5} (4 alike) : Scope
      Scope1 settings: TimeRange=auto  ShowLegends=on  MaxDataPoints=5000  SaveToWorkspace=off  SaveName=ScopeData6  YMin=-7.66216  YMax=6.81335  SampleTime=-1
      Scope2 settings: TimeRange=auto  MaxDataPoints=5000  SaveToWorkspace=off  SaveName=ScopeData7  YMin=-15.26187  YMax=29.35899  SampleTime=-1
      Scope3 settings: TimeRange=auto  ShowLegends=on  MaxDataPoints=5000  SaveToWorkspace=off  YMin=-53.89097  YMax=55.51694  SampleTime=-1
      Scope5 settings: TimeRange=auto  MaxDataPoints=5000  SaveToWorkspace=off  SaveName=ScopeData5  YMin=-1.81913  YMax=2.30438  SampleTime=-1
  Sum2 : Sum  Inputs=-++  SaturateOnIntegerOverflow=on  InputSameDT=on  OutDataTypeStr=Inherit: Same as first input
  Sum4 : Sum  Inputs=+++  SaturateOnIntegerOverflow=on  InputSameDT=on  OutDataTypeStr=Inherit: Same as first input
  Sum5 : Sum  Inputs=|+-  SaturateOnIntegerOverflow=on  InputSameDT=on  OutDataTypeStr=Inherit: Same as first input
  Uref : Outport
  Yref : Outport  Port=2
  wires:
  Sum5/1 -> Lo/1
  Cw/1 -> Sum5/2
  Integrator1/1 -> Cw/1, Aw/1, Gain5/1
  Sum4/1 -> Integrator1/1
  Aw/1 -> Sum4/3
  Lo/1 -> Sum4/1
  ro_previewed/1 -> Sum5/1, FIR Simpson 8/1(In1)
  Gain7/1 -> Mux2/1, Sum2/1
  Gain5/1 -> Mux2/2, Sum2/2
  FIR Simpson 8/1(Out1) -> Mux2/3, Sum2/3
  Ground/1 -> Sum4/2
  Sum2/1 -> Mux1/1, Uref/1  "Ta_ref"
  "ro_ref "/1 -> Mux1/3
  "fw "/1 -> Mux1/2
  Mesure/1(Out1) -> Scope5/1, Yref/1, Gain7/1
  Mux1/1 -> Scope2/1, ModèleVR/1(In1)
  ModèleVR/1(Out1) -> Scope1/1, Mesure/1(In1)
  Mux2/1 -> Scope3/1

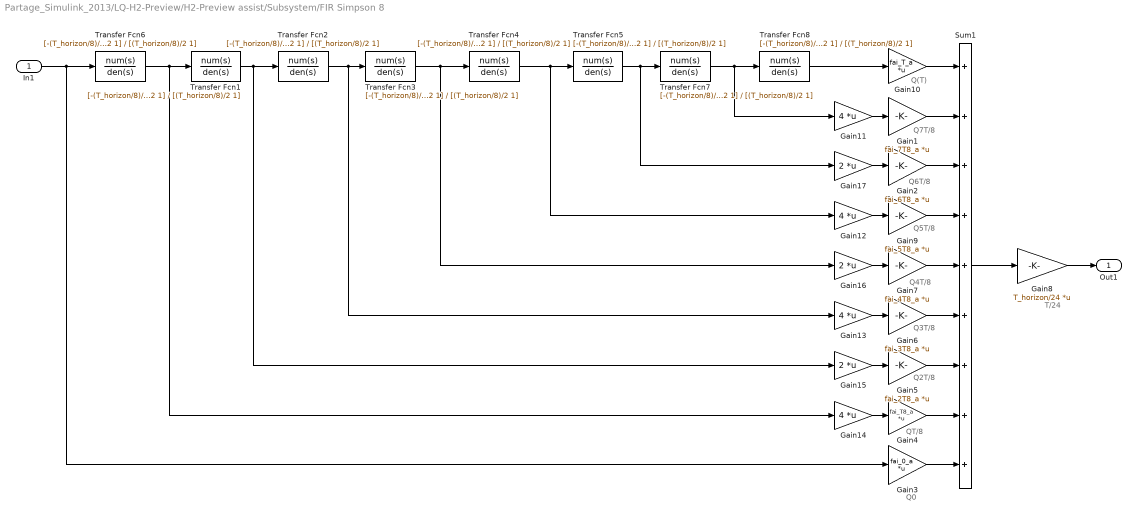
== system Partage_Simulink_2013/LQ-H2-Preview/H2-Preview assist/Subsystem/FIR Simpson 8 ==
  note: Q5T/8
  note: Q6T/8
  note: Q7T/8
  note: Q(T)
  note: T/24
  note: Q0
  note: QT/8
  note: Q2T/8
  note: Q3T/8
  note: Q4T/8
  In1 : Inport
  Gain1 : Gain  Gain=fai_7T8_a  Multiplication=Matrix(K*u)  SaturateOnIntegerOverflow=on  OutDataTypeStr=Inherit: Same as input  ParamDataTypeStr=Inherit: Same as input
  Gain10 : Gain  Gain=fai_T_a  Multiplication=Matrix(K*u)  SaturateOnIntegerOverflow=on  OutDataTypeStr=Inherit: Same as input  ParamDataTypeStr=Inherit: Same as input
  Gain{11..14} (4 alike) : Gain  Gain=4  Multiplication=Matrix(K*u)  SaturateOnIntegerOverflow=on  OutDataTypeStr=Inherit: Same as input  ParamDataTypeStr=Inherit: Same as input
  Gain15 : Gain  Gain=2  Multiplication=Matrix(K*u)  SaturateOnIntegerOverflow=on  OutDataTypeStr=Inherit: Same as input  ParamDataTypeStr=Inherit: Same as input
  Gain16 : Gain  Gain=2  Multiplication=Matrix(K*u)  SaturateOnIntegerOverflow=on  OutDataTypeStr=Inherit: Same as input  ParamDataTypeStr=Inherit: Same as input
  Gain17 : Gain  Gain=2  Multiplication=Matrix(K*u)  SaturateOnIntegerOverflow=on  OutDataTypeStr=Inherit: Same as input  ParamDataTypeStr=Inherit: Same as input
  Gain2 : Gain  Gain=fai_6T8_a  Multiplication=Matrix(K*u)  SaturateOnIntegerOverflow=on  OutDataTypeStr=Inherit: Same as input  ParamDataTypeStr=Inherit: Same as input
  Gain3 : Gain  Gain=fai_0_a  Multiplication=Matrix(K*u)  SaturateOnIntegerOverflow=on  OutDataTypeStr=Inherit: Same as input  ParamDataTypeStr=Inherit: Same as input
  Gain4 : Gain  Gain=fai_T8_a  Multiplication=Matrix(K*u)  SaturateOnIntegerOverflow=on  OutDataTypeStr=Inherit: Same as input  ParamDataTypeStr=Inherit: Same as input
  Gain5 : Gain  Gain=fai_2T8_a  Multiplication=Matrix(K*u)  SaturateOnIntegerOverflow=on  OutDataTypeStr=Inherit: Same as input  ParamDataTypeStr=Inherit: Same as input
  Gain6 : Gain  Gain=fai_3T8_a  Multiplication=Matrix(K*u)  SaturateOnIntegerOverflow=on  OutDataTypeStr=Inherit: Same as input  ParamDataTypeStr=Inherit: Same as input
  Gain7 : Gain  Gain=fai_4T8_a  Multiplication=Matrix(K*u)  SaturateOnIntegerOverflow=on  OutDataTypeStr=Inherit: Same as input  ParamDataTypeStr=Inherit: Same as input
  Gain8 : Gain  Gain=T_horizon/24  Multiplication=Matrix(K*u)  SaturateOnIntegerOverflow=on  OutDataTypeStr=Inherit: Same as input  ParamDataTypeStr=Inherit: Same as input
  Gain9 : Gain  Gain=fai_5T8_a  Multiplication=Matrix(K*u)  SaturateOnIntegerOverflow=on  OutDataTypeStr=Inherit: Same as input  ParamDataTypeStr=Inherit: Same as input
  Sum1 : Sum  Inputs=+++++++++  SaturateOnIntegerOverflow=on  InputSameDT=on  OutDataTypeStr=Inherit: Same as first input
  Transfer Fcn{1..8} (8 alike) : TransferFcn  Numerator=[-(T_horizon/8)/2 1]  Denominator=[(T_horizon/8)/2 1]
  Out1 : Outport
  wires:
  Transfer Fcn8/1 -> Gain10/1
  Sum1/1 -> Gain8/1
  Gain9/1 -> Sum1/4
  Gain2/1 -> Sum1/3
  Gain1/1 -> Sum1/2
  Gain10/1 -> Sum1/1
  Gain8/1 -> Out1/1
  Gain3/1 -> Sum1/9
  Gain7/1 -> Sum1/5
  Gain6/1 -> Sum1/6
  Gain5/1 -> Sum1/7
  Gain4/1 -> Sum1/8
  Gain11/1 -> Gain1/1
  Gain12/1 -> Gain9/1
  Gain13/1 -> Gain6/1
  Gain14/1 -> Gain4/1
  Gain15/1 -> Gain5/1
  Gain16/1 -> Gain7/1
  Gain17/1 -> Gain2/1
  Transfer Fcn7/1 -> Transfer Fcn8/1, Gain11/1
  Transfer Fcn5/1 -> Transfer Fcn7/1, Gain17/1
  Transfer Fcn4/1 -> Transfer Fcn5/1, Gain12/1
  Transfer Fcn3/1 -> Transfer Fcn4/1, Gain16/1
  Transfer Fcn2/1 -> Transfer Fcn3/1, Gain13/1
  Transfer Fcn1/1 -> Transfer Fcn2/1, Gain15/1
  Transfer Fcn6/1 -> Transfer Fcn1/1, Gain14/1
  In1/1 -> Transfer Fcn6/1, Gain3/1

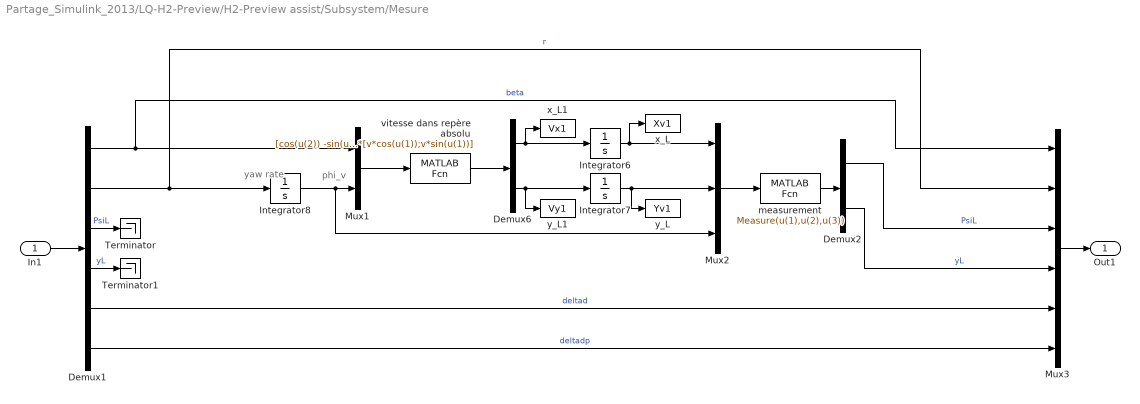
== system Partage_Simulink_2013/LQ-H2-Preview/H2-Preview assist/Subsystem/Mesure ==
  note: phi_v
  note: yaw rate
  In1 : Inport
  Demux1 : Demux  Outputs=6
  Demux2 : Demux  Outputs=2
  Demux6 : Demux  Outputs=2
  Integrator6 : Integrator  InitialCondition=EX0
  Integrator7 : Integrator  InitialCondition=EY0
  Integrator8 : Integrator  InitialCondition=EPHI0
  Mux1 : Mux  Inputs=2
  Mux2 : Mux  Inputs=3
  Mux3 : Mux  Inputs=6
  Terminator : Terminator
  Terminator1 : Terminator
  measurement : MATLABFcn  MATLABFcn=Measure(u(1),u(2),u(3))  OutputDimensions=2
  vitesse dans repère absolu : MATLABFcn  MATLABFcn=[cos(u(2)) -sin(u(2));sin(u(2)) cos(u(2)) ]*[v*cos(u(1));v*sin(u(1))]  OutputDimensions=2
  x_L : ToWorkspace  VariableName=Xv1  SampleTime=-1
  x_L1 : ToWorkspace  VariableName=Vx1  SampleTime=-1
  y_L : ToWorkspace  VariableName=Yv1  SampleTime=-1
  y_L1 : ToWorkspace  VariableName=Vy1  SampleTime=-1
  Out1 : Outport
  wires:
  Mux3/1 -> Out1/1
  In1/1 -> Demux1/1
  vitesse dans repère absolu/1 -> Demux6/1
  Integrator8/1 -> Mux2/3, Mux1/2
  Mux1/1 -> vitesse dans repère absolu/1
  Demux6/1 -> Integrator6/1, x_L1/1
  Demux6/2 -> y_L1/1, Integrator7/1
  Integrator6/1 -> Mux2/1, x_L/1
  Integrator7/1 -> y_L/1, Mux2/2
  Demux1/2 -> Mux3/2, Integrator8/1  "r"
  Demux1/1 -> Mux3/1, Mux1/1  "beta"
  Mux2/1 -> measurement/1
  measurement/1 -> Demux2/1
  Demux2/1 -> Mux3/3  "PsiL"
  Demux2/2 -> Mux3/4  "yL"
  Demux1/5 -> Mux3/5  "deltad"
  Demux1/6 -> Mux3/6  "deltadp"
  Demux1/3 -> Terminator/1  "PsiL"
  Demux1/4 -> Terminator1/1  "yL"

== system Partage_Simulink_2013/LQ-H2-Preview/H2-Preview assist/Subsystem/ModèleVR ==
  In1 : Inport
  Avr : Gain  Gain=Avr  Multiplication=Matrix(K*u)  SaturateOnIntegerOverflow=on  OutDataTypeStr=Inherit: Same as input  ParamDataTypeStr=Inherit: Same as input
  Bvr : Gain  Gain=Bvr  Multiplication=Matrix(K*u)  SaturateOnIntegerOverflow=on  OutDataTypeStr=Inherit: Same as input  ParamDataTypeStr=Inherit: Same as input
  Cvr : Gain  Gain=Cvr  Multiplication=Matrix(K*u)  SaturateOnIntegerOverflow=on  OutDataTypeStr=Inherit: Same as input  ParamDataTypeStr=Inherit: Same as input
  "Dvr " : Gain  Gain=Dvr  Multiplication=Matrix(K*u)  SaturateOnIntegerOverflow=on  OutDataTypeStr=Inherit: Same as input  ParamDataTypeStr=Inherit: Same as input
  Integrator2 : Integrator  ExternalReset=rising  InitialConditionSource=external
  Pulse Generator : DiscretePulseGenerator  PulseType=Time based  Period=5  PulseWidth=10
  Scope4 : Scope
      settings: TimeRange=auto  ShowLegends=on  MaxDataPoints=5000  SaveToWorkspace=off  SaveName=ScopeData8  YMin=-5.36347  YMax=6.60816  SampleTime=-1
  Sum1 : Sum  Inputs=|++  SaturateOnIntegerOverflow=on  InputSameDT=on  OutDataTypeStr=Inherit: Same as first input
  Sum3 : Sum  Inputs=++|  SaturateOnIntegerOverflow=on  InputSameDT=on  OutDataTypeStr=Inherit: Same as first input
  Out1 : Outport
  wires:
  In1/1 -> "Dvr "/1, Bvr/1
  Bvr/1 -> Sum1/1
  Avr/1 -> Sum1/2
  Sum1/1 -> Integrator2/1
  Integrator2/1 -> Avr/1, Cvr/1, Scope4/1
  Cvr/1 -> Sum3/2
  Sum3/1 -> Out1/1
  "Dvr "/1 -> Sum3/1
  [xc] -> Integrator2/3
  Pulse Generator/1 -> Integrator2/2
